simulink model "Copy_of_model_testslx_2015a"  (R2018b)
settings: Solver=ode3  StartTime=0.0  StopTime=100.0  FixedStep=0.01  RelTol=1e-3
values from neighbouring files (symbols this model uses):
  beta = params(1)    [model.m]
  g = 9.8105    [model.m]
  I = 0.0226    [model.m]
  K = params(3)    [model.m]
  K_lqr = lqr(A,B,Q,R)    [weryfikacja.m]
  tau = params(4)    [model.m]
  U = params(2)    [model.m]
  xep = [pi 0 0 0]    [weryfikacja.m]
settings Model: Creator=turgo  LastModifiedBy=Student
settings DataIOCC: ReturnWorkspaceOutputs=on
settings OptimizationCC: LifeSpan=inf
settings DebuggingCC: UnconnectedInputMsg=none  UnconnectedOutputMsg=none  UnconnectedLineMsg=none  SFExecutionAtInitializationDiag=none
settings HardwareCC: ProdBitPerSizeT=32  ProdBitPerPtrDiffT=32  ProdWordSize=32  ProdHWDeviceType=Specified
settings CodeAppCC: StateflowObjectComments=on

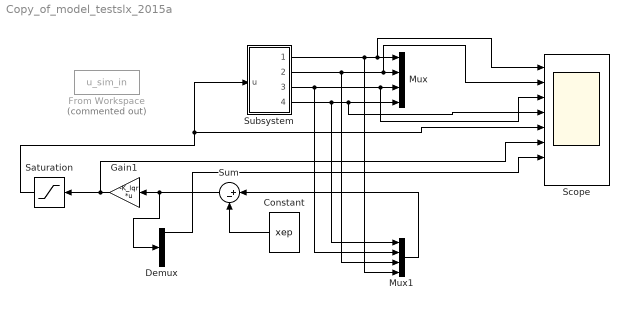
== system Copy_of_model_testslx_2015a ==
  Constant : Constant  Value=xep
  Demux : Demux
  From Workspace : FromWorkspace  Commented=on  VariableName=u_sim_in  SampleTime=0
  Gain1 : Gain  Gain=-K_lqr  Multiplication=Matrix(K*u) (u vector)
  Mux : Mux
  Mux1 : Mux
  Saturation : Saturate  UpperLimit=1  LowerLimit=-1
  Scope : Scope  NumInputPorts=8
  Subsystem : Subsystem
  Sum : Sum  Inputs=|+-
  wires:
  Subsystem/1(Out1) -> Mux1/4, Scope/1, Mux/1
  Subsystem/2(Out2) -> Mux1/3, Scope/2, Mux/2
  Subsystem/3(Out3) -> Mux1/2, Scope/3, Mux/3
  Subsystem/4(Out4) -> Mux1/1, Scope/4, Mux/4
  Gain1/1 -> Scope/6, Saturation/1
  Constant/1 -> Sum/2
  Sum/1 -> Demux/1, Gain1/1
  Saturation/1 -> Scope/5, Subsystem/1(u)
  Demux/1 -> Scope/7
  Mux1/1 -> Sum/1

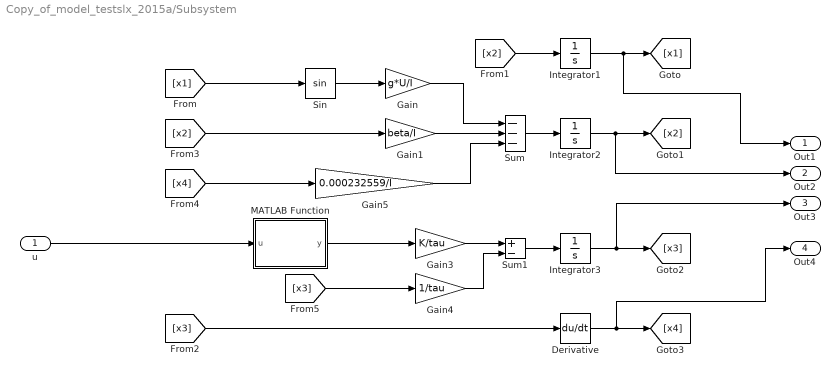
== system Copy_of_model_testslx_2015a/Subsystem ==
  u : Inport
  Derivative : Derivative
  Gain : Gain  Gain=g*U/I
  Gain1 : Gain  Gain=beta/I
  Gain3 : Gain  Gain=K/tau
  Gain4 : Gain  Gain=1/tau
  Gain5 : Gain  Gain=0.000232559/I
  Integrator1 : Integrator  InitialCondition=pi
  Integrator2 : Integrator
  Integrator3 : Integrator
  MATLAB Function : MATLAB Function  TreatAsAtomicUnit=on
  Sin : Trigonometry
  Sum : Sum  Inputs=---
  Sum1 : Sum  Inputs=+-
  Out1 : Outport
  Out2 : Outport  Port=2
  Out3 : Outport  Port=3
  Out4 : Outport  Port=4
  wires:
  [x1] -> Sin/1
  Integrator1/1 -> Out1/1, [x1]
  Sum/1 -> Integrator2/1
  Sum1/1 -> Integrator3/1
  Sin/1 -> Gain/1
  Gain/1 -> Sum/1
  Gain5/1 -> Sum/3
  Gain4/1 -> Sum1/2
  Gain3/1 -> Sum1/1
  [x2] -> Gain1/1
  [x2] -> Integrator1/1
  Integrator3/1 -> Out3/1, [x3]
  Gain1/1 -> Sum/2
  Integrator2/1 -> Out2/1, [x2]
  u/1 -> MATLAB Function/1(u)
  [x4] -> Gain5/1
  MATLAB Function/1(y) -> Gain3/1
  Derivative/1 -> Out4/1, [x4]
  [x3] -> Derivative/1
  [x3] -> Gain4/1

== matlab function Copy_of_model_testslx_2015a/Subsystem/MATLAB Function ==
  data: u input; y output
function y = fcn(u)

y = 211.6*u + 0.953;
